simulink model "Observerbased"  (R2019b)
settings: Solver=VariableStepAuto  StartTime=0.0  StopTime=50  RelTol=1e-3
values from neighbouring files (symbols this model uses):
  A = [-0.0964322196256 -1.97515329065 0.230033559961 0.526760251412 1.93131631395 -0.104255430496 0.375338290081 0.874573423921 -0.0824602195815 -0.23715349763 -0.0969848257774 -3.24166233906 ... (16 elements, 4x4)]    [Nord4stat_1in_6out.mat]    (also in Permutations.m = diag(v1))
  B = diag(v2)    [Permutations.m]    (also in obser_Main_Nodic.m = Bu)
  Bd = [-0.3308 0.7952 -0.7848 -1.2631]    [Nord4stat_1in_6out.mat]
  C = [1.16128585466 -0.574114782299 -0.79682308505 -0.802508498496 -0.119660607848 0.421861514188 -1.43156282695 0.618215593944 -0.346131117266 -0.341307508202 0.156479034542 -0.670980925729 ... (24 elements, 6x4)]    [Nord4stat_1in_6out.mat]
  Cz = [1 0 0 0]    [Nord4stat_1in_6out.mat]
  Dd = [0.6667 -1.3926 -1.3006 -0.605 -1.4886 0.5585]    [Nord4stat_1in_6out.mat]
  L = P\Y    [CongRPP.m]    (also in NFT.m; Permutations.m = I(a1(b1),:); cong.m; obser_BlockHadamard_new.m)
  state3 = [0,0,1,0]    [obser_Main_Nodic.m]
  y1 = eye(ny)    [obser_Main_Nodic.m]
  y2 = [0,0,0,0,0,0;0,0,0,0,0,0;0,0,0,0,0,0;0,0,0,0,0,0;0,0,0,0,1,0;0,0,0,0,0,0]    [obser_Main_Nodic.m]
undefined symbols (not defined in the file or in its folder): L0, L1, L3
libraries: dspswit3 x12
settings Model: Creator=Boxio  LastModifiedBy=wjl15

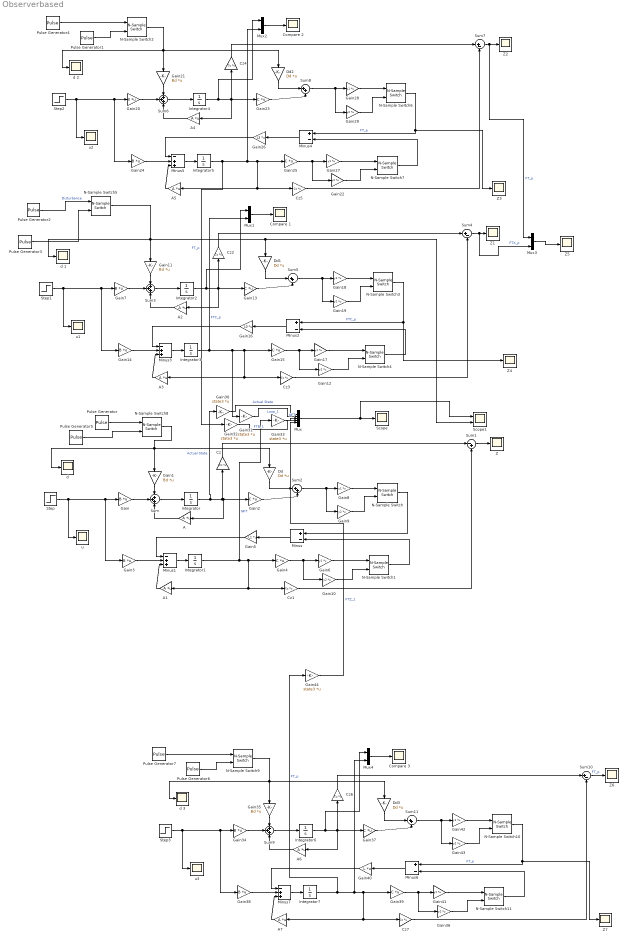
== system Observerbased ==
  A{,1..7} (8 alike) : Gain  Gain=A  Multiplication=Matrix(K*u)
  Compare 1 : Scope
  Compare 2 : Scope
  Compare 3 : Scope
  Cz{,1..7} (8 alike) : Gain  Gain=Cz  Multiplication=Matrix(K*u)
  Dd{,1..3} (4 alike) : Gain  Gain=Dd  Multiplication=Matrix(K*u)
  Gain{,3,7,14,20,24,34,38} (8 alike) : Gain  Gain=B  Multiplication=Matrix(K*u)
  Gain{1,11,21,35} (4 alike) : Gain  Gain=Bd  Multiplication=Matrix(K*u)
  Gain{9..10,12,19,22,29,36,43} (8 alike) : Gain  Gain=y2  Multiplication=Matrix(K*u)
  Gain{2,4,13,15,23,25,37,39} (8 alike) : Gain  Gain=C  Multiplication=Matrix(K*u)
  Gain16 : Gain  Gain=L0  Multiplication=Matrix(K*u)
  Gain{6,8,17..18,27..28,41..42} (8 alike) : Gain  Gain=y1  Multiplication=Matrix(K*u)
  Gain26 : Gain  Gain=L3  Multiplication=Matrix(K*u)
  Gain{30..33,44} (5 alike) : Gain  Gain=state3  Multiplication=Matrix(K*u)
  Gain40 : Gain  Gain=L  Multiplication=Matrix(K*u)
  Gain5 : Gain  Gain=L1  Multiplication=Matrix(K*u)
  Integrator{,1..7} (8 alike) : Integrator
  Minus{,2,4,6} (4 alike) : Sum  Inputs=+-
  Minus{1,3,5,7} (4 alike) : Sum  Inputs=-++
  Mux : Mux  Inputs=5
  Mux{1..4} (4 alike) : Mux  Inputs=2
  N-Sample Switch{,1,3..4,6..7,10..11} (8 alike) : dspswit3/N-Sample Switch  N=150  reset=off  TriggerType=Rising edge  Ts=0.1
      settings: SourceProductName=DSP System Toolbox  SourceProductBaseCode=DS
  N-Sample Switch{2,5,8..9} (4 alike) : dspswit3/N-Sample Switch  N=300  reset=off  TriggerType=Rising edge  Ts=0.1
      settings: SourceProductName=DSP System Toolbox  SourceProductBaseCode=DS
  Pulse Generator{,2,4,7} (4 alike) : DiscretePulseGenerator  PulseType=Time based  Amplitude=5  Period=15  PulseWidth=40  PhaseDelay=3
  Pulse Generator{1,3,5..6} (4 alike) : DiscretePulseGenerator  PulseType=Time based  Amplitude=0  Period=15  PulseWidth=40
  Scope : Scope
  Scope1 : Scope  NumInputPorts=2
  Step{,1..3} (4 alike) : Step  Time=0  After=0.1  SampleTime=0
  Sum{,3,6,9} (4 alike) : Sum  Inputs=3
  Sum1 : Sum  Inputs=|-+
  Sum10 : Sum  Inputs=|+-
  Sum{2,5,8,11} (4 alike) : Sum  Inputs=|++
  Sum4 : Sum  Inputs=|+-
  Sum7 : Sum  Inputs=|+-
  Z{,1..7} (8 alike) : Scope
  d {,1..3} (4 alike) : Scope
  u{,1..3} (4 alike) : Scope
  wires:
  Gain/1 -> Sum/2
  A/1 -> Sum/3
  Integrator/1 -> Gain30/1, A/1, Gain2/1, Cz/1  "Actual State"
  Sum/1 -> Integrator/1
  Gain1/1 -> Sum/1
  Gain2/1 -> Sum2/2
  Dd/1 -> Sum2/1
  Gain3/1 -> Minus1/2
  A1/1 -> Minus1/3
  Cz/1 -> Sum1/1
  Minus/1 -> Gain5/1
  Gain5/1 -> Minus1/1
  Minus1/1 -> Integrator1/1
  Integrator1/1 -> Gain33/1, A1/1, Cz1/1, Gain4/1  "NFT"
  Sum2/1 -> Gain9/1, Gain8/1
  Gain4/1 -> Gain10/1, Gain6/1
  Cz1/1 -> Sum1/2
  Sum1/1 -> Z/1
  Gain8/1 -> N-Sample Switch/1
  Gain9/1 -> N-Sample Switch/2
  N-Sample Switch/1 -> Minus/1
  Gain6/1 -> N-Sample Switch1/1
  Gain10/1 -> N-Sample Switch1/2
  N-Sample Switch1/1 -> Minus/2
  Step/1 -> u/1, Gain3/1, Gain/1
  Mux1/1 -> Compare 1/1
  A3/1 -> Minus3/3
  Minus2/1 -> Gain16/1
  Gain11/1 -> Sum3/1
  Gain17/1 -> N-Sample Switch4/1
  Gain16/1 -> Minus3/1
  Integrator3/1 -> A3/1, Cz3/1, Gain15/1, Gain31/1, Mux1/2  "FTC_p"
  Gain13/1 -> Sum5/2
  Gain15/1 -> Gain12/1, Gain17/1
  Gain14/1 -> Minus3/2
  Minus3/1 -> Integrator3/1
  Dd1/1 -> Sum5/1
  Integrator2/1 -> Mux1/1, A2/1, Gain13/1, Cz2/1
  Gain7/1 -> Sum3/2
  Cz3/1 -> Sum4/2
  Sum4/1 -> Mux3/2, Z1/1  "FTX_p"
  Step1/1 -> u1/1, Gain14/1, Gain7/1
  Cz2/1 -> Sum4/1
  Gain18/1 -> N-Sample Switch3/1
  Sum3/1 -> Integrator2/1
  A2/1 -> Sum3/3
  N-Sample Switch4/1 -> Minus2/2
  Gain12/1 -> N-Sample Switch4/2
  N-Sample Switch3/1 -> Z4/1, Minus2/1  "FTC_p"
  Sum5/1 -> Gain19/1, Gain18/1
  Gain19/1 -> N-Sample Switch3/2
  Mux2/1 -> Compare 2/1
  A5/1 -> Minus5/3
  Minus4/1 -> Gain26/1
  Gain21/1 -> Sum6/1
  Gain27/1 -> N-Sample Switch7/1
  Gain26/1 -> Minus5/1
  Gain23/1 -> Sum8/2
  Gain25/1 -> Gain22/1, Gain27/1
  Gain24/1 -> Minus5/2
  Minus5/1 -> Integrator5/1
  Dd2/1 -> Sum8/1
  Integrator4/1 -> Mux2/1, A4/1, Gain23/1, Cz4/1
  Gain20/1 -> Sum6/2
  Cz5/1 -> Sum7/2
  Sum7/1 -> Mux3/1, Z2/1  "FT_p"
  Step2/1 -> u2/1, Gain24/1, Gain20/1
  Cz4/1 -> Sum7/1
  Gain28/1 -> N-Sample Switch6/1
  Sum6/1 -> Integrator4/1
  A4/1 -> Sum6/3
  N-Sample Switch7/1 -> Minus4/2
  Gain22/1 -> N-Sample Switch7/2
  N-Sample Switch6/1 -> Z3/1, Minus4/1  "FT_p"
  Sum8/1 -> Gain29/1, Gain28/1
  Gain29/1 -> N-Sample Switch6/2
  Integrator5/1 -> Gain32/1, Mux2/2, A5/1, Cz5/1, Gain25/1  "FT_p"
  Gain30/1 -> Mux/1  "Actual State"
  Gain32/1 -> Mux/4  "FTB_1"
  Gain33/1 -> Mux/3  "NFT"
  Gain31/1 -> Mux/2  "Loop_1"
  Pulse Generator4/1 -> N-Sample Switch2/1
  N-Sample Switch2/1 -> Dd2/1, d 2/1, Gain21/1
  Pulse Generator1/1 -> N-Sample Switch2/2
  Pulse Generator2/1 -> N-Sample Switch5/1  "Disturbance"
  N-Sample Switch5/1 -> Scope1/2, Dd1/1, d 1/1, Gain11/1
  Pulse Generator3/1 -> N-Sample Switch5/2
  Pulse Generator/1 -> N-Sample Switch8/1
  N-Sample Switch8/1 -> Dd/1, "d "/1, Gain1/1
  Pulse Generator5/1 -> N-Sample Switch8/2
  Mux/1 -> Scope1/1, Scope/1
  Mux3/1 -> Z5/1
  N-Sample Switch11/1 -> Minus6/2
  Sum11/1 -> Gain43/1, Gain42/1
  Integrator6/1 -> Mux4/1, A6/1, Gain37/1, Cz6/1
  Mux4/1 -> Compare 3/1
  Pulse Generator6/1 -> N-Sample Switch9/2
  Gain36/1 -> N-Sample Switch11/2
  Gain37/1 -> Sum11/2
  Gain42/1 -> N-Sample Switch10/1
  Gain34/1 -> Sum9/2
  N-Sample Switch9/1 -> Dd3/1, d 3/1, Gain35/1
  Step3/1 -> u3/1, Gain38/1, Gain34/1
  Gain41/1 -> N-Sample Switch11/1
  Cz7/1 -> Sum10/2
  Gain39/1 -> Gain36/1, Gain41/1
  Gain43/1 -> N-Sample Switch10/2
  Integrator7/1 -> Gain44/1, Mux4/2, A7/1, Cz7/1, Gain39/1  "FT_p"
  Gain38/1 -> Minus7/2
  Dd3/1 -> Sum11/1
  Gain40/1 -> Minus7/1
  Gain35/1 -> Sum9/1
  Minus6/1 -> Gain40/1
  Cz6/1 -> Sum10/1
  Sum9/1 -> Integrator6/1
  Minus7/1 -> Integrator7/1
  A7/1 -> Minus7/3
  Pulse Generator7/1 -> N-Sample Switch9/1
  N-Sample Switch10/1 -> Z7/1, Minus6/1  "FT_p"
  Sum10/1 -> Z6/1  "FT_p"
  A6/1 -> Sum9/3
  Gain44/1 -> Mux/5  "FTZ_1"
